simulink model "backbone"  (R2022b)
settings: Solver=FixedStepDiscrete  StartTime=0.0  StopTime=2  FixedStep=0.000001  RelTol=1e-3
undefined symbols (not defined in the file or in its folder): DiscIntNeverNeededParam, flux, Motor_flux, Motor_Ld_Indctances, Motor_Lq_Indctances, Motor_Pn, Motor_Rs, Pn, switch_electronic_feedworward, Switch_SubsysCtrl, SysCurrentMax, SysVoltage, Ts
libraries: powerlib_extras x11, simulink x4, mcbcontrolslib x4, slpidlib x3, spsPermanentMagnetSynchronousMachineLib x2, spsDCVoltageSourceLib x2, spsGroundLib x1, eePmsmCurrentController x1, spsThreePhaseVIMeasurementLib x1, spsTwoLevelConverterLib x1, spsUniversalBridgeLib x1, spspowerguiLib x1
(part 1 of 3)
settings Model: DataDictionary=modelDictionary.sldd  PacingRate=0.018000  Creator=yll  LastModifiedBy=yll

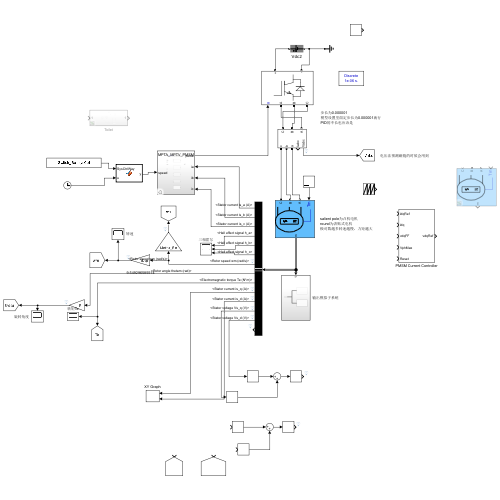
[thumbnail: Simulink's stored preview of the top-level diagram]
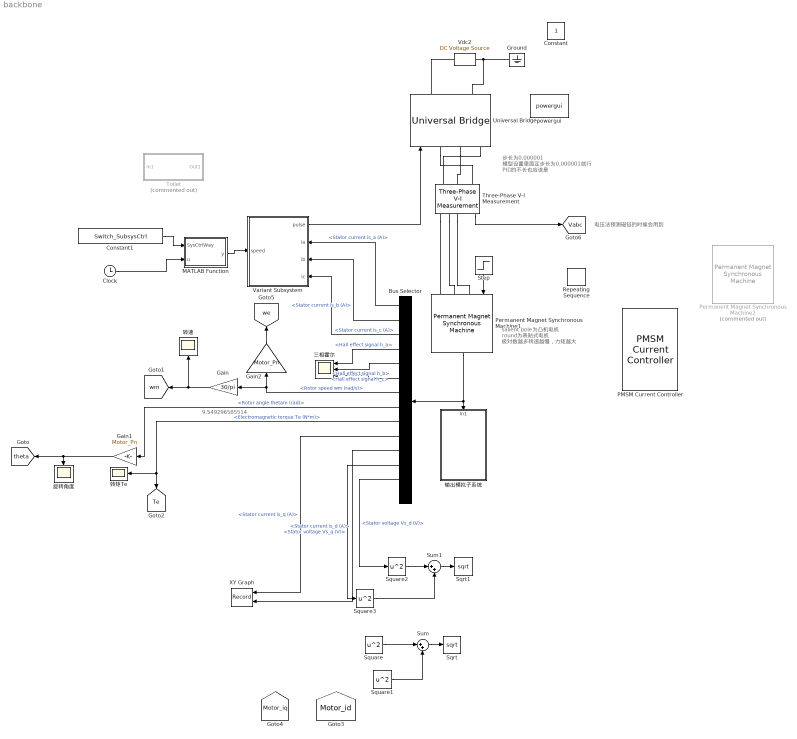
== system backbone ==
  note: 9.549296585514
  note: 电压法预测磁链的时候会用到
  note: salient pole为凸机电机
      | round为表贴式电机
      | 极对数越多转速越慢，力矩越大
  note: 步长为0.000001
      | 模型设置里面定步长为0.000001就行
      | PID的不长也应该是
  Bus Selector : BusSelector  OutputSignals=Stator current is_a (A),Stator current is_b (A),Stator current is_c (A),Hall effect signal h_a,Hall effect signal h_b,Hall effect signal h_c,Rotor speed wm (rad/s),Rotor angle thetam (rad),Electromagnetic torque Te (N*m),Stator current is_q (A),Stator current is_d (A),Stator voltage Vs_q (V),Stator voltage Vs_d (V),Electromagnetic torque Te (N*m)
  Clock : Clock
  Constant : Constant
  Constant1 : Constant  Value=Switch_SubsysCtrl
  Gain : Gain  Gain=30/pi
  Gain1 : Gain  Gain=Motor_Pn
  Gain2 : Gain  Gain=Motor_Pn
  Ground : spsGroundLib/Ground  LConnTagsString=a
  MATLAB Function : MATLAB Function  TreatAsAtomicUnit=on
  PMSM Current Controller : eePmsmCurrentController/PMSM Current Controller  Kp_id=1  Ki_id=100  Kaw_id=1  Kp_iq=1  Ki_iq=100  Kaw_iq=1  Ts=-1  Tsd=0.001  AxisPrio=Q-axis  ActZC=off  ActFF=on
      settings: LibrarySourceBlock=ee_sl_lib/PMSM Control/PMSM Current Controller
  Permanent Magnet Synchronous Machine1 : spsPermanentMagnetSynchronousMachineLib/Permanent Magnet Synchronous Machine  NbPhases=3  FluxDistribution=Sinusoidal  RotorType=Salient-pole  MechanicalLoad=Torque Tm  PresetModel=No  ShowDetailedParameters=on  MeasurementBus=off  Resistance=Motor_Rs  Inductance=8.5e-3  dqInductances=[Motor_Ld_Indctances Motor_Lq_Indctances]  La=Motor_Ld_Indctances  MachineConstant=Flux linkage established by magnets (V.s)  Flux=Motor_flux  VoltageCst=58.0416  TorqueCst=0.48  Flat=120  Mechanical=[0.003 0.008 Motor_Pn 0]  PolePairs=4  InitialConditions=[0,0, 0,0]  InitialConditions5ph=[0 0 0 0 0 0]  RefAngle=Aligned with phase A axis (original Park)  IterativeDiscreteModel=Trapezoidal robust  TsBlock=-1  TsPowergui=0
  Permanent Magnet Synchronous Machine2 : spsPermanentMagnetSynchronousMachineLib/Permanent Magnet Synchronous Machine  Commented=on  NbPhases=3  FluxDistribution=Sinusoidal  RotorType=Salient-pole  MechanicalLoad=Torque Tm  PresetModel=No  ShowDetailedParameters=on  MeasurementBus=off  Resistance=Motor_Rs  Inductance=8.5e-3  dqInductances=[Motor_Ld_Indctances Motor_Lq_Indctances]  La=Motor_Ld_Indctances  MachineConstant=Flux linkage established by magnets (V.s)  Flux=Motor_flux  VoltageCst=58.0416  TorqueCst=0.48  Flat=120  Mechanical=[0.003 0.008 Motor_Pn 0]  PolePairs=2  InitialConditions=[0,0, 0,0]  InitialConditions5ph=[0 0 0 0 0 0]  RefAngle=Aligned with phase A axis (original Park)  IterativeDiscreteModel=Trapezoidal robust  TsBlock=-1  TsPowergui=0
  Repeating Sequence : simulink/Sources/Repeating Sequence  rep_seq_t=[0 0.6 3]  rep_seq_y=[0 10 55.97]
  Sqrt : Sqrt
  Sqrt1 : Sqrt
  Square{,1..3} (4 alike) : Math  Operator=square
  Step : Step  Time=0.3  After=0  SampleTime=0
  Sum : Sum  Inputs=|++
  Sum1 : Sum  Inputs=|++
  Three-Phase V-I Measurement : spsThreePhaseVIMeasurementLib/Three-Phase V-I Measurement  VoltageMeasurement=phase-to-ground  SetLabelV=off  LabelV=Vabc  Vpu=off  VpuLL=off  CurrentMeasurement=yes  SetLabelI=off  LabelI=Iabc  Ipu=off  Pbase=100e6  Vbase=500e3  OutputType=Complex  PhasorSimulation=off  PSBequivalent=0
  Toilet : Subsystem  Commented=on
  Universal Bridge : spsUniversalBridgeLib/Universal Bridge  Arms=3  SnubberResistance=1e5  SnubberCapacitance=inf  Device=IGBT / Diodes  Ron=1e-3  Lon=0  ForwardVoltages="[  0  0  ]"  ForwardVoltage="[  0  0  ]"  GTOparameters=[ 10e-6 , 20e-6 ]  IGBTparameters=[ 1e-6 , 2e-6 ]  Measurements=None  Measurements_2=None  converterType=Rectifier
  Variant Subsystem : Subsystem  Variant=on
      settings: PortSchema="{\"entries\":[{\"content\":{\"sides\":[{\"content\":{\"connectorIds\":[\"In1\"]},\"type\":\"ConnectorPlacement.EquallySpacedRectSide\",\"uuid\":\"2e7849e6-0e6b-4177-ab4c-005e62b7a995\"},{\"content\":{\"connectorIds\":[\"Out1\",\"In2\",\"In3\",\"In4\"],\"side\":\"RIGHT\"},\"type\":\"ConnectorPlacement.EquallySpacedRectSide\",\"uuid\":\"63557eec-d5b5-4e2f-88ae-a2d5548ecb78\"},{\"content\":{\"connectorIds\":[],\"side\":\"TOP\"},\"type\":\"ConnectorPlacement.EquallySpacedRectSide\",\"uuid\":\"e5c96169-075b-4d07-a86b-1ba058334d10\"},{\"content\":{\"connectorIds\":[],\"side\":\"BOTTOM\"},\"type\":\"ConnectorPlacement.EquallySpacedRectSide\",\"uuid\":\"b7265cdc-8287-40f1-b4fb-8314bb99ac7b\"}]},\"type\":\"ConnectorPlacement.EquallySpacedConnector\",\"uuid\":\"3f47df4e-4e26-4395-afee-aeddf8227fe9\"}],\"packageUris\":[\"http://schema.mathworks.com/mf0/Connector/R2020b\"],\"version\":\"1.0\"}"
  Vdc2 : spsDCVoltageSourceLib/DC Voltage Source  Amplitude=SysVoltage  Measurements=None
  XY Graph : Record  FileSettingsInternal="{\"entries\":[{\"content\":{\"excelSettings\":{\"content\":{},\"type\":\"Streamout.ExcelSettings\"}},\"type\":\"Streamout.FileSettingStorage\",\"uuid\":\"9a52813c-0e76-4145-8ec9-bed97980991f\"}],\"packageUris\":[\"http://schema.mathworks.com/mf0/streamout_blocks/R2020a\"],\"version\":\"1.0\"}"  Layout=[1 1]  SignalsInternal="{\"entries\":[{\"content\":{\"signals\":[{\"content\":{\"blockPath\":[\"backbone/XY Graph\"],\"channel\":[],\"dimensions\":[1],\"domain\":\"backbone/XY Graph\",\"lineColor\":\"#a2142f\",\"plots\":[1],\"port\":1,\"sid\":[\"\"],\"signalID\":8996,\"signalName\":\"<Stator current is_q (A)>\"},\"type\":\"RecordBlkView.Signal\",\"uuid\":\"e11d3486-c8d0-4833-b26e-8d9d061e6f7c\"},{\"content\":{\"blockPath\":[\"backbone/XY Graph\"],\"channel\":[],\"dimensions\":[1],\"domain\":\"backbone/XY Graph\",\"lineColor\":\"#139fff\",\"plots\":[1],\"port\":2,\"sid\":[\"\"],\"signalID\":9000,\"signalName\":\"<Stator current is_d (A)>\"},\"type\":\"RecordBlkView.Signal\",\"uuid\":\"b0f723db-f625-4e0b-a689-0f7f588f8e97\"}]},\"type\":\"RecordBlkView.InputSignals\",\"uuid\":\"73730b23-746f-4a99-9d4b-303219e85664\"}],\"packageUris\":[\"http://schema.mathworks.com/mf0/streamout_blocks/R2020a\"],\"version\":\"1.0\"}"  VisualizationBindings="{\"xyplotplugin\":{\"info\":[{\"series\":[{\"bindingParametersList\":[{\"parameter\":\"X-Axis\",\"signalID\":8996,\"signalName\":\"<Stator current is_q (A)>\"},{\"parameter\":\"Y-Axis\",\"signalID\":9000,\"signalName\":\"<Stator current is_d (A)>\"}],\"seriesID\":62565}],\"subplotID\":1}]}}"  CompatibilityTag=XY
  powergui : spspowerguiLib/powergui  Priority=1  SimulationMode=Discrete  SampleTime=1e-6  frequency=60  Iterations=50  frequencyindice=0  Pbase=100e6  ErrMax=1e-4  UnitsV=kV  UnitsW=MW  buscounter=0  FunctionMessages=off  echomessages=off  EnableUseOfTLC=off  CurrentSourceSwitches=off  DisableSnubberDevices=off  DisableRonSwitches=off  DisableVfSwitches=off  DisplayEquations=off  AutomaticDiscreteSolvers=off  SolverType=Tustin/Backward Euler (TBE)  Interpol=off  ExternalGateDelay=off  methode=off  Ts=10  x0status=blocks  SPID=off  SwTol=0  HookPort=off  NonlinearTolerance=1e-4  nMaxIteration=100  ContinueOnMaxIteration=off  RestoreLinks=warning  ResistiveCurrentMeasurement=off  Frange=[0:2:500]  Ylog=off  Xlog=on  ShowGrid=off  save=off  variable=ZData  structure=current_abc  ZoomFFT=off  StartTime=0.1  cycles=1  DisplayStyle=1  fundamental=1  FreqAxis=off  MaxFrequency=100  frequencyindicesteady=1  RmsSteady=1  display=off
  三相霍尔 : Scope  NumInputPorts=3
  旋转角度 : Scope
  转矩Te : Scope
  转速 : Scope
  输出模拟子系统 : Subsystem
  tag scope: Motor_id=global, Motor_iq=global, Te=global, Vabc=global, theta=global, we=global, wm=global
  wires:
  Gain1/1 -> 旋转角度/1, [theta]
  Bus Selector/6 -> 三相霍尔/3  "<Hall effect signal h_c>"
  Bus Selector/4 -> 三相霍尔/1  "<Hall effect signal h_a>"
  Bus Selector/5 -> 三相霍尔/2  "<Hall effect signal h_b>"
  Gain/1 -> [wm], 转速/1
  Bus Selector/8 -> Gain1/1  "<Rotor angle thetam (rad)>"
  Bus Selector/7 -> Gain2/1, Gain/1  "<Rotor speed wm (rad/s)>"
  Permanent Magnet Synchronous Machine1/1 -> Bus Selector/1, 输出模拟子系统/1(In1)
  Variant Subsystem/1(pulse) -> Universal Bridge/1
  Gain2/1 -> [we]
  Three-Phase V-I Measurement/1 -> [Vabc]
  Bus Selector/9 -> [Te], 转矩Te/1  "<Electromagnetic torque Te (N*m)>"
  Bus Selector/1 -> Variant Subsystem/2(ia)  "<Stator current is_a (A)>"
  Bus Selector/2 -> Variant Subsystem/3(ib)  "<Stator current is_b (A)>"
  Bus Selector/3 -> Variant Subsystem/4(ic)  "<Stator current is_c (A)>"
  Square/1 -> Sum/1
  Square1/1 -> Sum/2
  Sum/1 -> Sqrt/1
  Square2/1 -> Sum1/1
  Sum1/1 -> Sqrt1/1
  Square3/1 -> Sum1/2
  Bus Selector/12 -> Square3/1  "<Stator voltage Vs_q (V)>"
  Bus Selector/13 -> Square2/1  "<Stator voltage Vs_d (V)>"
  Step/1 -> Permanent Magnet Synchronous Machine1/1
  Bus Selector/10 -> XY Graph/1  "<Stator current is_q (A)>"
  Bus Selector/11 -> XY Graph/2  "<Stator current is_d (A)>"
  Clock/1 -> MATLAB Function/2(u)
  MATLAB Function/1(y) -> Variant Subsystem/1(speed)
  Constant1/1 -> MATLAB Function/1(SysCtrlWay)
  connections:
  Vdc2/RConn1 -- Universal Bridge/RConn1
  Vdc2/LConn1 -- Universal Bridge/RConn2 -- Ground/LConn1
  Universal Bridge/LConn1 -- Three-Phase V-I Measurement/LConn1
  Universal Bridge/LConn2 -- Three-Phase V-I Measurement/LConn2
  Universal Bridge/LConn3 -- Three-Phase V-I Measurement/LConn3
  Three-Phase V-I Measurement/RConn1 -- Permanent Magnet Synchronous Machine1/LConn1
  Three-Phase V-I Measurement/RConn2 -- Permanent Magnet Synchronous Machine1/LConn2
  Three-Phase V-I Measurement/RConn3 -- Permanent Magnet Synchronous Machine1/LConn3

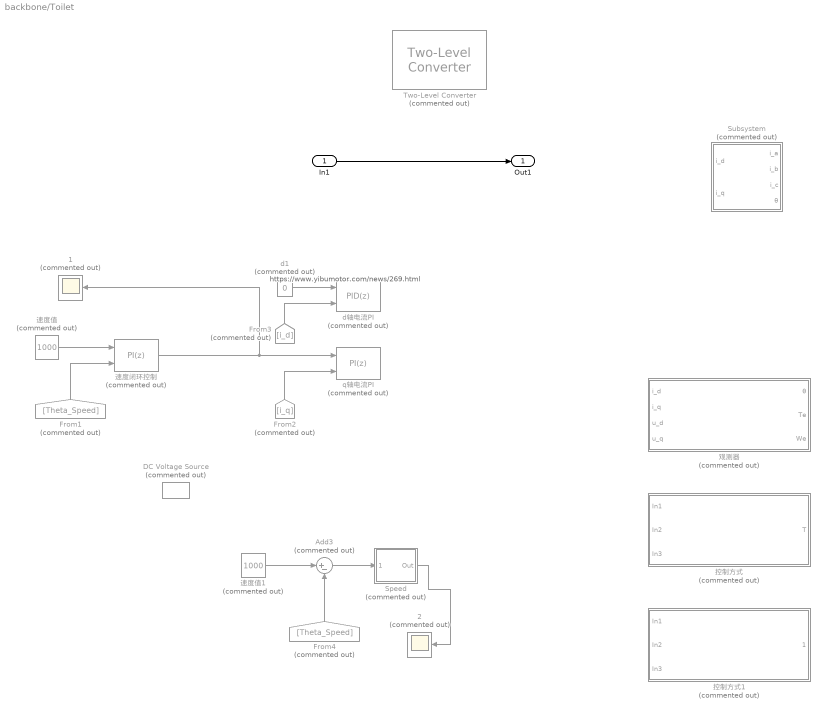
== system backbone/Toilet ==
  note: https://www.yibumotor.com/news/269.html
  In1 : Inport
  " 1" : Scope  Commented=on
  " 2" : Scope  Commented=on
  Add3 : Sum  Commented=on  Inputs=|+-
  DC Voltage Source : spsDCVoltageSourceLib/DC Voltage Source  Commented=on  Amplitude=311  Measurements=None
  From1 : From  Commented=on  GotoTag=Theta_Speed
  From2 : From  Commented=on  GotoTag=i_q
  From3 : From  Commented=on  GotoTag=i_d
  From4 : From  Commented=on  GotoTag=Theta_Speed
  Speed : Subsystem  Commented=on  AncestorBlock=|  DialogController=POWERSYS.PowerSysDialog  mask(Discrete PI Controller){C=1, Mu=1, q=200, Par_Limits=[1000 -1000], Init=0, Ts=0.000001}
      | powerlib_extras/Discrete 
      | Control Blocks/Discrete
      | PI Controller
      mask prompts: C "Gain (c):"; Mu "Gain (Mu):"; q "Gain (q)"; Par_Limits "Output limits: [ Upper   Lower ]"; Init "Output initial value:"; Ts "Sample time:"
      mask help: This block implements a discrete PI controller.
      mask init:
      | UpperLimit=Par_Limits(1);
      | LowerLimit=Par_Limits(2);
      | power_initmask();
      settings: LibrarySourceBlock=|
      | powerlib_extras/Discrete
      | Control Blocks/Discrete
      | PI Controller
      mask Help: This block is part of a subset of blocks in the Extras library that does not have documentation associated with it, other than the block mask description.
      mask Display: disp('SMC');
  Subsystem : Subsystem  Commented=on
  Two-Level Converter : spsTwoLevelConverterLib/Two-Level Converter  Commented=on  ModelType=Switching devices  Ron=1e-3  Rs=1e6  Cs=inf  Vforward=[0,0]  Ron_Diode=1e-3  Rs_Diode=1e6  Cs_Diode=inf  Vf_Diode=1e-3  Rs_CurrentSource=inf  Ron_ACsource=1e-3
      settings: LibrarySourceBlock=sps_lib/Power Electronics/Two-Level Converter
  d1 : Constant  Commented=on  Value=0
  d轴电流PI : slpidlib/PID Controller (2DOF)  Commented=on  Controller=PID  Form=Parallel  TimeDomain=Discrete-time  UseExternalTs=off  SampleTime=-1  IntegratorMethod=Forward Euler  FilterMethod=Forward Euler  ControllerParametersSource=internal  P=16.4  I=5750  UseKiTs=off  D=0  N=100  UseFilter=on  b=1  c=1  TunerSelectOption=Transfer Function Based (PID Tuner App)  InitialConditionSource=internal  InitialConditionForIntegrator=0  InitialConditionForFilter=0  DifferentiatorICPrevScaledInput=0  ExternalReset=none  TrackingMode=off  Kt=1  LimitOutput=off  SatLimitsSource=internal  UpperSaturationLimit=inf  LowerSaturationLimit=-inf  LinearizeAsGain=off  AntiWindupMode=none  Kb=1  LimitIntegrator=off  UpperIntegratorSaturationLimit=inf  LowerIntegratorSaturationLimit=-inf  POutMin=[]  POutMax=[]  IOutMin=[]  IOutMax=[]  DOutMin=[]  DOutMax=[]  NOutMin=[]  NOutMax=[]  bOutMin=[]  bOutMax=[]  cOutMin=[]  cOutMax=[]  SumOutMin=[]  SumOutMax=[]  SaturationOutMin=[]  SaturationOutMax=[]  PParamMin=[]  PParamMax=[]  IParamMin=[]  IParamMax=[]  DParamMin=[]  DParamMax=[]  NParamMin=[]  NParamMax=[]  bParamMin=[]  bParamMax=[]  cParamMin=[]  cParamMax=[]  KbParamMin=[]  KbParamMax=[]  KtParamMin=[]  KtParamMax=[]  KbOutMin=[]  KbOutMax=[]  KtOutMin=[]  KtOutMax=[]  IntegratorOutMin=[]  IntegratorOutMax=[]  FilterOutMin=[]  FilterOutMax=[]  SumI1OutMin=[]  SumI1OutMax=[]  SumI2OutMin=[]  SumI2OutMax=[]  SumI3OutMin=[]  SumI3OutMax=[]  SumI4OutMin=[]  SumI4OutMax=[]  SumDOutMin=[]  SumDOutMax=[]  Sum1OutMin=[]  Sum1OutMax=[]  Sum2OutMin=[]  Sum2OutMax=[]  Sum3OutMin=[]  Sum3OutMax=[]  DifferentiatorOutMin=[]  DifferentiatorOutMax=[]  FilterDiffOutCoefMin=[]  FilterDiffOutCoefMax=[]  ReciprocalOutMin=[]  ReciprocalOutMax=[]  SumDenOutMin=[]  SumDenOutMax=[]  SumNumOutMin=[]  SumNumOutMax=[]  DivideOutMin=[]  DivideOutMax=[]  UdiffTsProdOutMin=[]  UdiffTsProdOutMax=[]  NTsProdOutMin=[]  NTsProdOutMax=[]  UintegralTsProdOutMin=[]  UintegralTsProdOutMax=[]  UngainTsProdOutMin=[]  UngainTsProdOutMax=[]  ClampingZeroOutDataTypeStr=Inherit: Inherit via back propagation  ClampingZeroOutMin=[]  ClampingZeroOutMax=[]  FilterDenConstantOutDataTypeStr=Inherit: Inherit via back propagation  FilterDenConstantOutMin=[]  FilterDenConstantOutMax=[]  PCopyOutDataTypeStr=Inherit: Inherit via back propagation  PCopyOutMin=[]  PCopyOutMax=[]  NCopyOutDataTypeStr=Inherit: Inherit via back propagation  NCopyOutMin=[]  NCopyOutMax=[]  IntegratorContinuousStateAttributes=''  IntegratorStateMustResolveToSignalObject=off  IntegratorRTWStateStorageClass=Auto  FilterContinuousStateAttributes=''  FilterStateMustResolveToSignalObject=off  FilterRTWStateStorageClass=Auto  ParallelPVariant=InternalParameters  IdealPVariant=Disabled  IVariant=InternalParameters  DVariant=InternalParameters  bVariant=InternalParameters  cVariant=InternalParameters  IntegratorVariant=Discrete  SatVariant=Disabled  AWVariant=Passthrough  PCopyVariant=Disabled  TRVariant=Disabled  FdbkBlocksVariant=Forward  IdealPFdbkVariant=Disabled  SatFdbkVariant=Disabled  DerivativeFilterVariant=ForwardEulerFilter  NVariant=InternalParameters  NCopyVariant=Disabled  FilterICVariant=InternalICsFilter  IntegratorICVariant=InternalICs  ExternalResetVariant=Disabled  TRSumVariant=Passthrough  SumFdbkVariant=Disabled  SumVariant=Sum_PID  TsampFilterVariant=InternalTs  TsampNgainVariant=Passthrough  TsampIntegralVariant=Passthrough  ExternalSaturationOutDataTypeStr=Inherit: Same as second input
  q轴电流PI : slpidlib/PID Controller (2DOF)  Commented=on  Controller=PI  Form=Parallel  TimeDomain=Discrete-time  UseExternalTs=off  SampleTime=0.000001  IntegratorMethod=Forward Euler  FilterMethod=Forward Euler  ControllerParametersSource=internal  P=16.4  I=5750  UseKiTs=off  D=0  N=100  UseFilter=on  b=1  c=1  TunerSelectOption=Transfer Function Based (PID Tuner App)  InitialConditionSource=internal  InitialConditionForIntegrator=0  InitialConditionForFilter=0  DifferentiatorICPrevScaledInput=0  ExternalReset=none  TrackingMode=off  Kt=1  LimitOutput=off  SatLimitsSource=internal  UpperSaturationLimit=inf  LowerSaturationLimit=-inf  LinearizeAsGain=off  AntiWindupMode=none  Kb=1  LimitIntegrator=off  UpperIntegratorSaturationLimit=inf  LowerIntegratorSaturationLimit=-inf  POutMin=[]  POutMax=[]  IOutMin=[]  IOutMax=[]  DOutMin=[]  DOutMax=[]  NOutMin=[]  NOutMax=[]  bOutMin=[]  bOutMax=[]  cOutMin=[]  cOutMax=[]  SumOutMin=[]  SumOutMax=[]  SaturationOutMin=[]  SaturationOutMax=[]  PParamMin=[]  PParamMax=[]  IParamMin=[]  IParamMax=[]  DParamMin=[]  DParamMax=[]  NParamMin=[]  NParamMax=[]  bParamMin=[]  bParamMax=[]  cParamMin=[]  cParamMax=[]  KbParamMin=[]  KbParamMax=[]  KtParamMin=[]  KtParamMax=[]  KbOutMin=[]  KbOutMax=[]  KtOutMin=[]  KtOutMax=[]  IntegratorOutMin=[]  IntegratorOutMax=[]  FilterOutMin=[]  FilterOutMax=[]  SumI1OutMin=[]  SumI1OutMax=[]  SumI2OutMin=[]  SumI2OutMax=[]  SumI3OutMin=[]  SumI3OutMax=[]  SumI4OutMin=[]  SumI4OutMax=[]  SumDOutMin=[]  SumDOutMax=[]  Sum1OutMin=[]  Sum1OutMax=[]  Sum2OutMin=[]  Sum2OutMax=[]  Sum3OutMin=[]  Sum3OutMax=[]  DifferentiatorOutMin=[]  DifferentiatorOutMax=[]  FilterDiffOutCoefMin=[]  FilterDiffOutCoefMax=[]  ReciprocalOutMin=[]  ReciprocalOutMax=[]  SumDenOutMin=[]  SumDenOutMax=[]  SumNumOutMin=[]  SumNumOutMax=[]  DivideOutMin=[]  DivideOutMax=[]  UdiffTsProdOutMin=[]  UdiffTsProdOutMax=[]  NTsProdOutMin=[]  NTsProdOutMax=[]  UintegralTsProdOutMin=[]  UintegralTsProdOutMax=[]  UngainTsProdOutMin=[]  UngainTsProdOutMax=[]  ClampingZeroOutDataTypeStr=Inherit: Inherit via back propagation  ClampingZeroOutMin=[]  ClampingZeroOutMax=[]  FilterDenConstantOutDataTypeStr=Inherit: Inherit via back propagation  FilterDenConstantOutMin=[]  FilterDenConstantOutMax=[]  PCopyOutDataTypeStr=Inherit: Inherit via back propagation  PCopyOutMin=[]  PCopyOutMax=[]  NCopyOutDataTypeStr=Inherit: Inherit via back propagation  NCopyOutMin=[]  NCopyOutMax=[]  IntegratorContinuousStateAttributes=''  IntegratorStateMustResolveToSignalObject=off  IntegratorRTWStateStorageClass=Auto  FilterContinuousStateAttributes=''  FilterStateMustResolveToSignalObject=off  FilterRTWStateStorageClass=Auto  ParallelPVariant=InternalParameters  IdealPVariant=Disabled  IVariant=InternalParameters  DVariant=Disabled  bVariant=InternalParameters  cVariant=Disabled  IntegratorVariant=Discrete  SatVariant=Disabled  AWVariant=Passthrough  PCopyVariant=Disabled  TRVariant=Disabled  FdbkBlocksVariant=Forward  IdealPFdbkVariant=Disabled  SatFdbkVariant=Disabled  DerivativeFilterVariant=Disabled  NVariant=Disabled  NCopyVariant=Disabled_SignalSpec  FilterICVariant=Disabled  IntegratorICVariant=InternalICs  ExternalResetVariant=Disabled  TRSumVariant=Passthrough  SumFdbkVariant=Disabled  SumVariant=Sum_PI  TsampFilterVariant=InternalTs  TsampNgainVariant=Passthrough  TsampIntegralVariant=Passthrough  ExternalSaturationOutDataTypeStr=Inherit: Same as second input
  控制方式 : Subsystem  Commented=on  Variant=on
  控制方式1 : Subsystem  Commented=on  Variant=on
  观测器 : Subsystem  Commented=on  Variant=on
  速度值 : Constant  Commented=on  Value=1000
  速度值1 : Constant  Commented=on  Value=1000
  速度闭环控制 : slpidlib/PID Controller (2DOF)  Commented=on  Controller=PI  Form=Parallel  TimeDomain=Discrete-time  UseExternalTs=off  SampleTime=0.000001  IntegratorMethod=Forward Euler  FilterMethod=Forward Euler  ControllerParametersSource=internal  P=0.7  I=5  UseKiTs=off  D=0  N=100  UseFilter=on  b=1  c=1  TunerSelectOption=Transfer Function Based (PID Tuner App)  InitialConditionSource=internal  InitialConditionForIntegrator=0  InitialConditionForFilter=0  DifferentiatorICPrevScaledInput=0  ExternalReset=none  TrackingMode=off  Kt=1  LimitOutput=off  SatLimitsSource=internal  UpperSaturationLimit=inf  LowerSaturationLimit=-inf  LinearizeAsGain=off  AntiWindupMode=none  Kb=1  LimitIntegrator=off  UpperIntegratorSaturationLimit=inf  LowerIntegratorSaturationLimit=-inf  POutMin=[]  POutMax=[]  IOutMin=[]  IOutMax=[]  DOutMin=[]  DOutMax=[]  NOutMin=[]  NOutMax=[]  bOutMin=[]  bOutMax=[]  cOutMin=[]  cOutMax=[]  SumOutMin=[]  SumOutMax=[]  SaturationOutMin=[]  SaturationOutMax=[]  PParamMin=[]  PParamMax=[]  IParamMin=[]  IParamMax=[]  DParamMin=[]  DParamMax=[]  NParamMin=[]  NParamMax=[]  bParamMin=[]  bParamMax=[]  cParamMin=[]  cParamMax=[]  KbParamMin=[]  KbParamMax=[]  KtParamMin=[]  KtParamMax=[]  KbOutMin=[]  KbOutMax=[]  KtOutMin=[]  KtOutMax=[]  IntegratorOutMin=[]  IntegratorOutMax=[]  FilterOutMin=[]  FilterOutMax=[]  SumI1OutMin=[]  SumI1OutMax=[]  SumI2OutMin=[]  SumI2OutMax=[]  SumI3OutMin=[]  SumI3OutMax=[]  SumI4OutMin=[]  SumI4OutMax=[]  SumDOutMin=[]  SumDOutMax=[]  Sum1OutMin=[]  Sum1OutMax=[]  Sum2OutMin=[]  Sum2OutMax=[]  Sum3OutMin=[]  Sum3OutMax=[]  DifferentiatorOutMin=[]  DifferentiatorOutMax=[]  FilterDiffOutCoefMin=[]  FilterDiffOutCoefMax=[]  ReciprocalOutMin=[]  ReciprocalOutMax=[]  SumDenOutMin=[]  SumDenOutMax=[]  SumNumOutMin=[]  SumNumOutMax=[]  DivideOutMin=[]  DivideOutMax=[]  UdiffTsProdOutMin=[]  UdiffTsProdOutMax=[]  NTsProdOutMin=[]  NTsProdOutMax=[]  UintegralTsProdOutMin=[]  UintegralTsProdOutMax=[]  UngainTsProdOutMin=[]  UngainTsProdOutMax=[]  ClampingZeroOutDataTypeStr=Inherit: Inherit via back propagation  ClampingZeroOutMin=[]  ClampingZeroOutMax=[]  FilterDenConstantOutDataTypeStr=Inherit: Inherit via back propagation  FilterDenConstantOutMin=[]  FilterDenConstantOutMax=[]  PCopyOutDataTypeStr=Inherit: Inherit via back propagation  PCopyOutMin=[]  PCopyOutMax=[]  NCopyOutDataTypeStr=Inherit: Inherit via back propagation  NCopyOutMin=[]  NCopyOutMax=[]  IntegratorContinuousStateAttributes=''  IntegratorStateMustResolveToSignalObject=off  IntegratorRTWStateStorageClass=Auto  FilterContinuousStateAttributes=''  FilterStateMustResolveToSignalObject=off  FilterRTWStateStorageClass=Auto  ParallelPVariant=InternalParameters  IdealPVariant=Disabled  IVariant=InternalParameters  DVariant=Disabled  bVariant=InternalParameters  cVariant=Disabled  IntegratorVariant=Discrete  SatVariant=Disabled  AWVariant=Passthrough  PCopyVariant=Disabled  TRVariant=Disabled  FdbkBlocksVariant=Forward  IdealPFdbkVariant=Disabled  SatFdbkVariant=Disabled  DerivativeFilterVariant=Disabled  NVariant=Disabled  NCopyVariant=Disabled_SignalSpec  FilterICVariant=Disabled  IntegratorICVariant=InternalICs  ExternalResetVariant=Disabled  TRSumVariant=Passthrough  SumFdbkVariant=Disabled  SumVariant=Sum_PI  TsampFilterVariant=InternalTs  TsampNgainVariant=Passthrough  TsampIntegralVariant=Passthrough  ExternalSaturationOutDataTypeStr=Inherit: Same as second input
  Out1 : Outport
  wires:
  In1/1 -> Out1/1
  From2/1 -> q轴电流PI/2
  d1/1 -> d轴电流PI/1
  From4/1 -> Add3/2
  From1/1 -> 速度闭环控制/2
  From3/1 -> d轴电流PI/2
  速度闭环控制/1 -> q轴电流PI/1, " 1"/1
  速度值1/1 -> Add3/1
  Add3/1 -> Speed/1(Error)
  速度值/1 -> 速度闭环控制/1
  Speed/1(Out) -> " 2"/1

== system backbone/Variant Subsystem ==
  note: 1) Add Subsystem or Model blocks as valid variant choices.
      | 2) You cannot connect blocks at this level. At simulation, connectivity is automatically
      | determined, based on the active variant and port name matching.
  speed : Inport
  ia : Inport  Port=2
  ib : Inport  Port=3
  ic : Inport  Port=4
  BangBang_PMSM : Subsystem  VariantControl=Switch_SubsysCtrl==2
  DTC_PMSM : Subsystem  VariantControl=Switch_SubsysCtrl==3
  DTC_SVPWM_PMSM : Subsystem  VariantControl=Switch_SubsysCtrl==4
  MPTA_MPTV_PMSM : Subsystem  VariantControl=Switch_SubsysCtrl==5
  SMC_OR_PID : Subsystem  VariantControl=Switch_SubsysCtrl==0|Switch_SubsysCtrl==1
  pulse : Outport

== system backbone/输出模拟子系统 ==
  In1 : Inport
  clark和park变换模拟 : Subsystem  Commented=on
  磁链模拟 : Subsystem
  wires:
  In1/1 -> 磁链模拟/1(In1), clark和park变换模拟/1(In1)

== system backbone/Toilet/Speed ==
  Error : Inport  SampleTime=Ts
  1/D : Gain  Gain=1/(1.5*Pn*flux/0.003)  SaturateOnIntegerOverflow=on  SampleTime=Ts  OutDataTypeStr=Inherit: Same as input  ParamDataTypeStr=Inherit: Same as input
  Discrete Derivative : simulink/Discrete/Discrete Derivative  gainval=1.0  ICPrevScaledInput=0.0  OutMin=[]  OutMax=[]  OutDataType=fixdt(1, 16)  OutScaling=2^-10  DoSatur=off
  Discrete-Time Integrator : DiscreteIntegrator  InitialCondition=0.001  SampleTime=Ts  ICPrevOutput=DiscIntNeverNeededParam  ICPrevScaledInput=DiscIntNeverNeededParam
  Kp1 : Gain  Gain=q  SaturateOnIntegerOverflow=on  SampleTime=Ts  OutDataTypeStr=Inherit: Same as input  ParamDataTypeStr=Inherit: Same as input
  Kp2 : Gain  Gain=Mu  SaturateOnIntegerOverflow=on  SampleTime=Ts  OutDataTypeStr=Inherit: Same as input  ParamDataTypeStr=Inherit: Same as input
  Kp3 : Gain  Gain=C  SaturateOnIntegerOverflow=on  SampleTime=Ts  OutDataTypeStr=Inherit: Same as input  ParamDataTypeStr=Inherit: Same as input
  Kp4 : Gain  Gain=C  SaturateOnIntegerOverflow=on  SampleTime=Ts  OutDataTypeStr=Inherit: Same as input  ParamDataTypeStr=Inherit: Same as input
  Nr->wm : Gain  Gain=pi/30  SaturateOnIntegerOverflow=on  SampleTime=Ts  OutDataTypeStr=Inherit: Same as input  ParamDataTypeStr=Inherit: Same as input
  Saturation2 : Saturate  UpperLimit=UpperLimit  LowerLimit=LowerLimit  SampleTime=Ts
  Sign : Signum
  Sum1 : Sum  InputSameDT=on  SaturateOnIntegerOverflow=on  SampleTime=Ts  OutDataTypeStr=Inherit: Same as first input
  Sum2 : Sum  Inputs=++-  InputSameDT=on  SaturateOnIntegerOverflow=on  SampleTime=Ts  OutDataTypeStr=Inherit: Same as first input
  Out : Outport  SampleTime=Ts  InitialOutput=0
  wires:
  Kp4/1 -> Sum1/1
  Saturation2/1 -> Out/1
  Discrete Derivative/1 -> Kp3/1, Sum1/2
  Sum2/1 -> Discrete-Time Integrator/1
  Error/1 -> Nr->wm/1
  Kp1/1 -> Sum2/1
  Sign/1 -> Kp2/1
  Sum1/1 -> Sign/1, Kp1/1
  Kp2/1 -> Sum2/2
  Kp3/1 -> Sum2/3
  1/D/1 -> Saturation2/1
  Discrete-Time Integrator/1 -> 1/D/1
  Nr->wm/1 -> Discrete Derivative/1, Kp4/1

== system backbone/Toilet/Subsystem ==
  i_a : Inport
  i_b : Inport  Port=2
  i_c : Inport  Port=3
  θ : Inport  Port=4
  Model : ModelReference  ModelNameDialog=ParkTran.slx  SimulationMode=Normal  ModelReferenceVersion=1.9
  Model1 : ModelReference  ModelNameDialog=ClarkTran.slx  SimulationMode=Normal  ModelReferenceVersion=1.13
  三相电流3 : Scope  NumInputPorts=3
  三相电流4 : Scope  NumInputPorts=2
  三相电流5 : Scope  NumInputPorts=2
  i_d : Outport
  i_q : Outport  Port=2
  wires:
  Model1/1 -> 三相电流4/1, Model/1
  i_b/1 -> Model1/2, 三相电流3/2
  Model1/2 -> 三相电流4/2, Model/2
  Model/1 -> i_d/1, 三相电流5/1
  Model/2 -> i_q/1, 三相电流5/2
  i_a/1 -> Model1/1, 三相电流3/1
  i_c/1 -> Model1/3, 三相电流3/3
  θ/1 -> Model/3

== system backbone/Toilet/控制方式 ==
  note: 1) Add Subsystem or Model blocks as valid variant choices.
      | 2) You cannot connect blocks at this level. At simulation, connectivity is automatically
      | determined, based on the active variant and port name matching.
  In1 : Inport
  In2 : Inport  Port=2
  In3 : Inport  Port=3
  DTC : ModelReference  ModelNameDialog=testmodel2.slx  VariantControl=true  ModelReferenceVersion=1.7
  FOC : ModelReference  DisableCoverage=on  ModelNameDialog=testmodel1.slx  VariantControl=false  ModelReferenceVersion=1.6
  T : Outport

== system backbone/Toilet/控制方式1 ==
  note: 1) Add Subsystem or Model blocks as valid variant choices.
      | 2) You cannot connect blocks at this level. At simulation, connectivity is automatically
      | determined, based on the active variant and port name matching.
  In1 : Inport
  In2 : Inport  Port=2
  In3 : Inport  Port=3
  PWM : ModelReference  DisableCoverage=on  ModelNameDialog=testmodel1.slx  VariantControl=false  ModelReferenceVersion=1.6
  SPWM : ModelReference  ModelNameDialog=testmodel2.slx  VariantControl=false  ModelReferenceVersion=1.7
  SVPWM : ModelReference  ModelNameDialog=testmodel2.slx  VariantControl=true  ModelReferenceVersion=1.7
  1 : Outport

== system backbone/Toilet/观测器 ==
  note: 1) Add Subsystem or Model blocks as valid variant choices.
      | 2) You cannot connect blocks at this level. At simulation, connectivity is automatically
      | determined, based on the active variant and port name matching.
  i_d : Inport
  i_q : Inport  Port=2
  u_d : Inport  Port=3
  u_q : Inport  Port=4
  Extended Kalman Filter : ModelReference  ModelNameDialog=testmodel2.slx  VariantControl=vm_Observer_Switch==2  ModelReferenceVersion=1.7
  Stationary coordinate system SMC αβ : ModelReference  ModelNameDialog=testmodel2.slx  VariantControl=vm_Observer_Switch==3  ModelReferenceVersion=1.7
  Synchronous rotating coordinate system SMC dq : ModelReference  DisableCoverage=on  ModelNameDialog=testmodel1.slx  VariantControl=vm_Observer_Switch==1  ModelReferenceVersion=1.6
  θ : Outport
  Te : Outport  Port=2
  We : Outport  Port=3

== system backbone/Variant Subsystem/BangBang_PMSM ==
  ia : Inport
  ib : Inport  Port=2
  ic : Inport  Port=3
  speed : Inport  Port=4
  Constant : Constant  Value=0
  Model1 : ModelReference  ModelNameDialog=InvParkTran.slx  SimulationMode=Normal  ModelReferenceVersion=1.8
  Model2 : ModelReference  ModelNameDialog=BangBang.slx  SimulationMode=Normal  ModelReferenceVersion=1.26
  Speed : Subsystem  AncestorBlock=|  DialogController=POWERSYS.PowerSysDialog  mask(Discrete PI Controller){Kpw=0.073, Kiw=0, Ba=0, Par_Limits=[50*sqrt(2) -50*sqrt(2)], Init=0, Ts=Ts}
      | powerlib_extras/Discrete 
      | Control Blocks/Discrete
      | PI Controller
      mask prompts: Kpw "Proportional gain (Kp):"; Kiw "Integral gain (Ki):"; Ba "feedback gain (Ba)"; Par_Limits "Output limits: [ Upper   Lower ]"; Init "Output initial value:"; Ts "Sample time:"
      mask help: This block implements a discrete PI controller.
      mask init:
      | UpperLimit=Par_Limits(1);
      | LowerLimit=Par_Limits(2);
      | power_initmask();
      settings: LibrarySourceBlock=|
      | powerlib_extras/Discrete
      | Control Blocks/Discrete
      | PI Controller
      mask Help: This block is part of a subset of blocks in the Extras library that does not have documentation associated with it, other than the block mask description.
      mask Display: disp('PI');
  Sum : Sum  Inputs=|+-
  pulse : Outport
  wires:
  speed/1 -> Sum/1
  [we] -> Sum/2
  Sum/1 -> Speed/1(Error)
  [theta] -> Model1/3
  ia/1 -> Model2/1
  ic/1 -> Model2/3
  ib/1 -> Model2/2
  Speed/1(Out) -> Model1/2
  Model1/1 -> Model2/4
  Model1/2 -> Model2/5
  Model2/1 -> pulse/1
  Constant/1 -> Model1/1

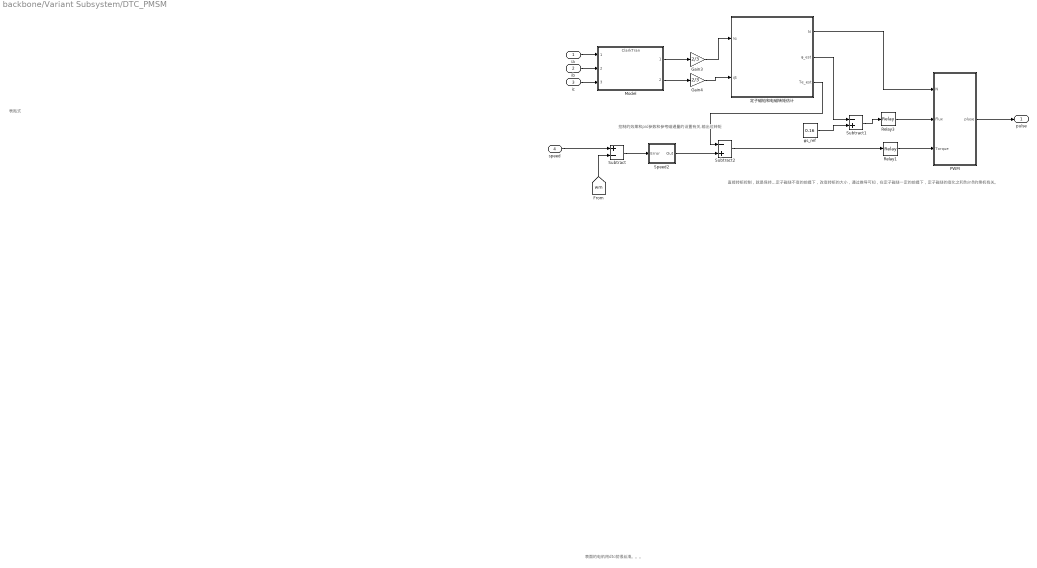
== system backbone/Variant Subsystem/DTC_PMSM ==
  note: 表贴式
  note: 控制的效果和pid参数和参考磁通量的设置有关,输出位转矩
  note: 直接转矩控制，就是保持定子磁链不变的前提下，改变转矩的大小，通过推导可知，在定子磁链一定的前提下，定子磁链的变化之和θsinθ的乘机有关。
  note: 表面的电机用dtc就很丝滑。。。
  ia : Inport
  ib : Inport  Port=2
  ic : Inport  Port=3
  speed : Inport  Port=4
  Gain3 : Gain  Gain=2/3
  Gain4 : Gain  Gain=2/3
  Model : ModelReference  ModelNameDialog=ClarkTran.slx  SimulationMode=Normal  ModelReferenceVersion=1.13
  PWM : Subsystem
  Relay1 : Relay  OnSwitchValue=0.00002  OffSwitchValue=-0.00002
  Relay3 : Relay  OnSwitchValue=0.00002  OffSwitchValue=-0.00002  InputProcessing=Columns as channels (frame based)
  Speed2 : Subsystem  AncestorBlock=|  DialogController=POWERSYS.PowerSysDialog  mask(Discrete PI Controller){Kpw=0.0114, Kiw=0.019, Ba=0, Par_Limits=[33.49 -33.49], Init=0, Ts=1e-6}
      | powerlib_extras/Discrete 
      | Control Blocks/Discrete
      | PI Controller
      mask prompts: Kpw "Proportional gain (Kp):"; Kiw "Integral gain (Ki):"; Ba "feedback gain (Ba)"; Par_Limits "Output limits: [ Upper   Lower ]"; Init "Output initial value:"; Ts "Sample time:"
      mask help: This block implements a discrete PI controller.
      mask init:
      | UpperLimit=Par_Limits(1);
      | LowerLimit=Par_Limits(2);
      | power_initmask();
      settings: LibrarySourceBlock=|
      | powerlib_extras/Discrete
      | Control Blocks/Discrete
      | PI Controller
      mask Help: This block is part of a subset of blocks in the Extras library that does not have documentation associated with it, other than the block mask description.
      mask Display: disp('PI');
  Subtract : Sum  Inputs=+-
  Subtract1 : Sum  Inputs=-+
  Subtract2 : Sum  Inputs=-+
  φs_ref : Constant  Value=0.16  VectorParams1D=off  SampleTime=Ts
  定子磁链和电磁转矩估计 : Subsystem  Variant=on
  pulse : Outport
  wires:
  ib/1 -> Model/2
  [wm] -> Subtract/2
  Relay1/1 -> PWM/3(Torque)
  Relay3/1 -> PWM/2(Flux)
  PWM/1(pluse) -> pulse/1
  Subtract1/1 -> Relay3/1
  φs_ref/1 -> Subtract1/2
  speed/1 -> Subtract/1
  Subtract2/1 -> Relay1/1
  定子磁链和电磁转矩估计/2(φ_est) -> Subtract1/1
  定子磁链和电磁转矩估计/1(N) -> PWM/1(N)
  ia/1 -> Model/1
  ic/1 -> Model/3
  定子磁链和电磁转矩估计/3(Te_est) -> Subtract2/1
  Speed2/1(Out) -> Subtract2/2
  Subtract/1 -> Speed2/1(Error)
  Model/2 -> Gain4/1
  Gain4/1 -> 定子磁链和电磁转矩估计/2(iβ)
  Model/1 -> Gain3/1
  Gain3/1 -> 定子磁链和电磁转矩估计/1(Iα)

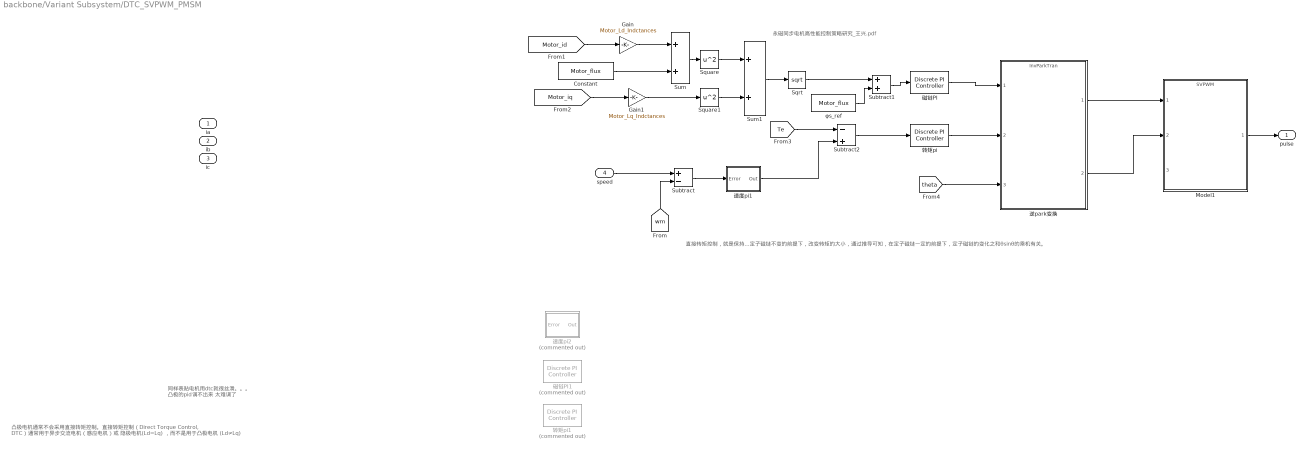
== system backbone/Variant Subsystem/DTC_SVPWM_PMSM ==
  note: 凸极电机通常不会采用直接转矩控制。直接转矩控制（Direct Torque Control, DTC）通常用于异步交流电机（感应电机）或 隐极电机(Ld=Lq) ，而不是用于凸极电机 (Ld≠Lq)
  note: 永磁同步电机高性能控制策略研究_王兴.pdf
  note: 直接转矩控制，就是保持定子磁链不变的前提下，改变转矩的大小，通过推导可知，在定子磁链一定的前提下，定子磁链的变化之和θsinθ的乘机有关。
  note: 同样表贴电机用dtc就很丝滑。。。
      | 凸极的pid调不出来 太难调了
  ia : Inport
  ib : Inport  Port=2
  ic : Inport  Port=3
  speed : Inport  Port=4
  Constant : Constant  Value=Motor_flux
  Gain : Gain  Gain=Motor_Ld_Indctances
  Gain1 : Gain  Gain=Motor_Lq_Indctances
  Model1 : ModelReference  ModelNameDialog=SVPWM.slx  SimulationMode=Normal  ModelReferenceVersion=1.9
  Sqrt : Sqrt
  Square : Math  Operator=square
  Square1 : Math  Operator=square
  Subtract : Sum  Inputs=+-
  Subtract1 : Sum
  Subtract2 : Sum  Inputs=-+
  Sum : Sum
  Sum1 : Sum
  φs_ref : Constant  Value=Motor_flux  SampleTime=Ts
  磁链PI : powerlib_extras/Discrete  Control Blocks/Discrete PI Controller  Kp=0.8  Ki=4  Par_Limits=[2 -2]  Init=0  Ts=Ts
  磁链PI1 : powerlib_extras/Discrete  Control Blocks/Discrete PI Controller  Commented=on  Kp=0.8  Ki=4  Par_Limits=[2 -2]  Init=0  Ts=Ts
  转矩pi : powerlib_extras/Discrete  Control Blocks/Discrete PI Controller  Kp=0.75  Ki=0.1  Par_Limits=[1000000 -1000000]  Init=0  Ts=Ts
  转矩pi1 : powerlib_extras/Discrete  Control Blocks/Discrete PI Controller  Commented=on  Kp=0.75  Ki=0.1  Par_Limits=[10000 -10000]  Init=0  Ts=Ts
  逆park变换 : ModelReference  ModelNameDialog=InvParkTran.slx  SimulationMode=Normal  ModelReferenceVersion=1.8
  速度pi1 : Subsystem  AncestorBlock=|  DialogController=POWERSYS.PowerSysDialog  mask(Discrete PI Controller){Kpw=0.0114, Kiw=0.019, Ba=0, Par_Limits=[34 -34], Init=0, Ts=Ts}
      | powerlib_extras/Discrete 
      | Control Blocks/Discrete
      | PI Controller
      mask prompts: Kpw "Proportional gain (Kp):"; Kiw "Integral gain (Ki):"; Ba "feedback gain (Ba)"; Par_Limits "Output limits: [ Upper   Lower ]"; Init "Output initial value:"; Ts "Sample time:"
      mask help: This block implements a discrete PI controller.
      mask init:
      | UpperLimit=Par_Limits(1);
      | LowerLimit=Par_Limits(2);
      | power_initmask();
      settings: LibrarySourceBlock=|
      | powerlib_extras/Discrete
      | Control Blocks/Discrete
      | PI Controller
      mask Help: This block is part of a subset of blocks in the Extras library that does not have documentation associated with it, other than the block mask description.
      mask Display: disp('PI');
  速度pi2 : Subsystem  Commented=on  AncestorBlock=|  DialogController=POWERSYS.PowerSysDialog  mask(Discrete PI Controller){Kpw=0.5, Kiw=120, Ba=0, Par_Limits=[1600 -1600], Init=0, Ts=Ts}
      | powerlib_extras/Discrete 
      | Control Blocks/Discrete
      | PI Controller
      mask prompts: Kpw "Proportional gain (Kp):"; Kiw "Integral gain (Ki):"; Ba "feedback gain (Ba)"; Par_Limits "Output limits: [ Upper   Lower ]"; Init "Output initial value:"; Ts "Sample time:"
      mask help: This block implements a discrete PI controller.
      mask init:
      | UpperLimit=Par_Limits(1);
      | LowerLimit=Par_Limits(2);
      | power_initmask();
      settings: LibrarySourceBlock=|
      | powerlib_extras/Discrete
      | Control Blocks/Discrete
      | PI Controller
      mask Help: This block is part of a subset of blocks in the Extras library that does not have documentation associated with it, other than the block mask description.
      mask Display: disp('PI');
  pulse : Outport
  wires:
  [Te] -> Subtract2/1
  Subtract/1 -> 速度pi1/1(Error)
  Sqrt/1 -> Subtract1/1
  speed/1 -> Subtract/1
  φs_ref/1 -> Subtract1/2
  [wm] -> Subtract/2
  Model1/1 -> pulse/1
  Subtract2/1 -> 转矩pi/1
  Subtract1/1 -> 磁链PI/1
  Sum/1 -> Square/1
  Constant/1 -> Sum/2
  [Motor_id] -> Gain/1
  [Motor_iq] -> Gain1/1
  Square1/1 -> Sum1/2
  Square/1 -> Sum1/1
  Sum1/1 -> Sqrt/1
  磁链PI/1 -> 逆park变换/1
  转矩pi/1 -> 逆park变换/2
  [theta] -> 逆park变换/3
  逆park变换/1 -> Model1/1
  逆park变换/2 -> Model1/2
  速度pi1/1(Out) -> Subtract2/2
  Gain/1 -> Sum/1
  Gain1/1 -> Square1/1

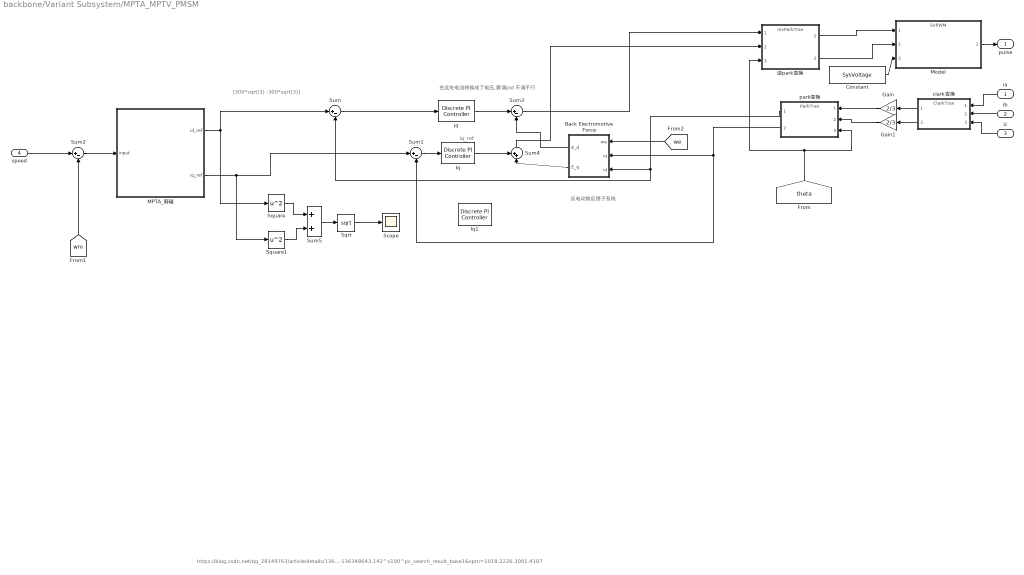
== system backbone/Variant Subsystem/MPTA_MPTV_PMSM ==
  note: [300*sqrt(3) -300*sqrt(3)]
  note: https://blog.csdn.net/qq_28149763/article/details/136348643?ops_request_misc=&request_id=&biz_id=102&utm_term=%E8%B6%85%E5%89%8D%E8%A7%92%E8%AE%A1%E7%AE%97MPTA&utm_medium=distribute.pc_search_result.none-task-blog-2~all~sobaiduweb~default-2-136348643.142^v100^pc_search_result_base1&spm=1018.2226.3001.4187
  note: iq_ref
  note: 反电动势反馈子系统
  note: 在此处电流转换成了电压,要调pid 不调不行
  ia : Inport
  ib : Inport  Port=2
  ic : Inport  Port=3
  speed : Inport  Port=4
  Back Electromotive Force : Subsystem
  Constant : Constant  Value=SysVoltage
  Gain : Gain  Gain=2/3
  Gain1 : Gain  Gain=2/3
  Id : powerlib_extras/Discrete  Control Blocks/Discrete PI Controller  Kp=50  Ki=0  Par_Limits=[300*sqrt(3) -300*sqrt(3)]  Init=0  Ts=Ts
  Iq : powerlib_extras/Discrete  Control Blocks/Discrete PI Controller  Kp=50  Ki=0  Par_Limits=[300*sqrt(3) -300*sqrt(3)]  Init=0  Ts=Ts
  Iq1 : powerlib_extras/Discrete  Control Blocks/Discrete PI Controller  Kp=0.1  Ki=0  Par_Limits=[SysVoltage*0.9*sqrt(3) -SysVoltage*0.9*sqrt(3)]  Init=0  Ts=Ts
  MPTA_弱磁 : Subsystem  Variant=on
  Model : ModelReference  ModelNameDialog=SVPWM.slx  SimulationMode=Normal  ModelReferenceVersion=1.9
  Scope : Scope
  Sqrt : Sqrt
  Square : Math  Operator=square
  Square1 : Math  Operator=square
  Sum{,1..3} (4 alike) : Sum  Inputs=|+-
  Sum4 : Sum  Inputs=++|
  Sum5 : Sum
  clark变换 : ModelReference  ModelNameDialog=ClarkTran.slx  SimulationMode=Normal  ModelReferenceVersion=1.13
  park变换 : ModelReference  ModelNameDialog=ParkTran.slx  SimulationMode=Normal  ModelReferenceVersion=1.9
  逆park变换 : ModelReference  ModelNameDialog=InvParkTran.slx  SimulationMode=Normal  ModelReferenceVersion=1.8
  pulse : Outport
  wires:
  Sum3/1 -> 逆park变换/1
  park变换/2 -> Back Electromotive Force/2(iq), Sum1/2
  Sum4/1 -> 逆park变换/2
  Back Electromotive Force/1(E_d) -> Sum3/2
  clark变换/2 -> Gain1/1
  ia/1 -> clark变换/1
  Square/1 -> Sum5/1
  Sqrt/1 -> Scope/1
  ic/1 -> clark变换/3
  ib/1 -> clark变换/2
  Sum1/1 -> Iq/1
  clark变换/1 -> Gain/1
  Iq/1 -> Sum4/1
  [theta] -> park变换/3, 逆park变换/3
  Back Electromotive Force/2(E_q) -> Sum4/2
  Id/1 -> Sum3/1
  Sum/1 -> Id/1
  park变换/1 -> Sum/2, Back Electromotive Force/3(id)
  [wm] -> Sum2/2
  逆park变换/2 -> Model/2
  speed/1 -> Sum2/1
  Square1/1 -> Sum5/2
  Model/1 -> pulse/1
  逆park变换/1 -> Model/1
  Gain/1 -> park变换/1
  Sum5/1 -> Sqrt/1
  [we] -> Back Electromotive Force/1(we)
  Gain1/1 -> park变换/2
  Sum2/1 -> MPTA_弱磁/1(input)
  MPTA_弱磁/2(iq_ref) -> Square1/1, Sum1/1
  MPTA_弱磁/1(id_ref) -> Sum/1, Square/1
  Constant/1 -> Model/3

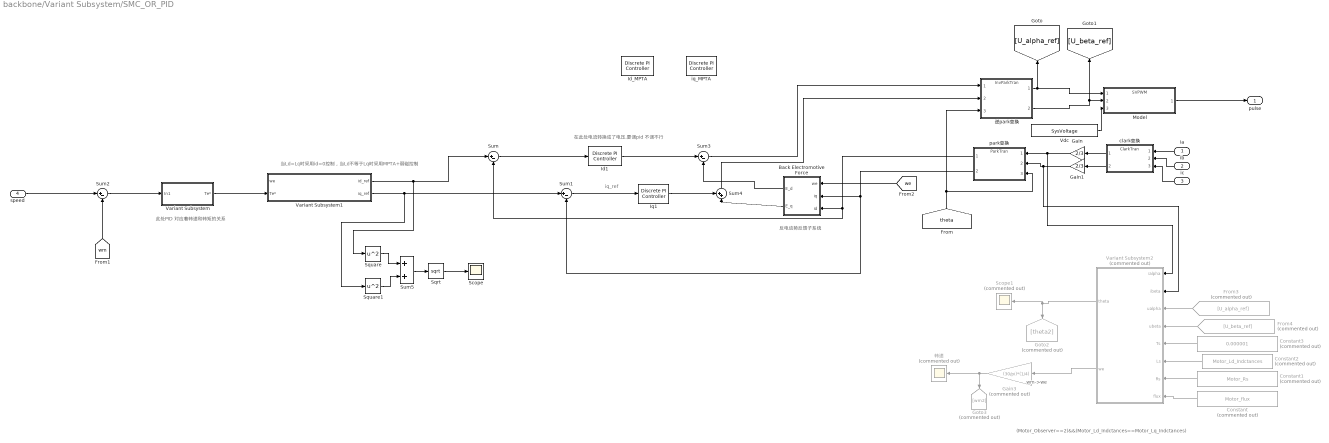
== system backbone/Variant Subsystem/SMC_OR_PID ==
  note: 当Ld=Lq时采用id=0控制，当Ld不等于Lq时采用MPTA+弱磁控制
  note: 此处PID 对应着转速和转矩的关系
  note: (Motor_Observer==2)&&(Motor_Ld_Indctances==Motor_Lq_Indctances)
  note: 在此处电流转换成了电压,要调pid 不调不行
  note: wm->we
  note: iq_ref
  note: 反电动势反馈子系统
  ia : Inport
  ib : Inport  Port=2
  ic : Inport  Port=3
  speed : Inport  Port=4
  Back Electromotive Force : Subsystem
  Constant : Constant  Commented=on  Value=Motor_flux
  Constant1 : Constant  Commented=on  Value=Motor_Rs
  Constant2 : Constant  Commented=on  Value=Motor_Ld_Indctances
  Constant3 : Constant  Commented=on  Value=0.000001
  From3 : From  Commented=on  GotoTag=U_alpha_ref
  From4 : From  Commented=on  GotoTag=U_beta_ref
  Gain : Gain  Gain=2/3
  Gain1 : Gain  Gain=2/3
  Gain3 : Gain  Commented=on  Gain=(30/pi)*(1/4)
  Goto2 : Goto  Commented=on  GotoTag=theta2
  Goto3 : Goto  Commented=on  GotoTag=wm2
  Id1 : powerlib_extras/Discrete  Control Blocks/Discrete PI Controller  Kp=133  Ki=0  Par_Limits=[SysVoltage*sqrt(3) -SysVoltage*sqrt(3)]  Init=0  Ts=1e-5
  Id_MPTA : powerlib_extras/Discrete  Control Blocks/Discrete PI Controller  Kp=50  Ki=250  Par_Limits=[4000 -4000]  Init=0  Ts=Ts
  Iq1 : powerlib_extras/Discrete  Control Blocks/Discrete PI Controller  Kp=133  Ki=0  Par_Limits=[SysVoltage*sqrt(3) -SysVoltage*sqrt(3)]  Init=0  Ts=1e-5
  Model : ModelReference  ModelNameDialog=SVPWM.slx  SimulationMode=Normal  ModelReferenceVersion=1.9
  Scope : Scope
  Scope1 : Scope  Commented=on
  Sqrt : Sqrt
  Square : Math  Operator=square
  Square1 : Math  Operator=square
  Sum{,1..3} (4 alike) : Sum  Inputs=|+-
  Sum4 : Sum  Inputs=++|
  Sum5 : Sum
  Variant Subsystem : Subsystem  Variant=on
  Variant Subsystem1 : Subsystem  Variant=on
  Variant Subsystem2 : Subsystem  Commented=on  Variant=on
  Vdc : Constant  Value=SysVoltage
  clark变换 : ModelReference  ModelNameDialog=ClarkTran.slx  SimulationMode=Normal  ModelReferenceVersion=1.13
  iq_MPTA : powerlib_extras/Discrete  Control Blocks/Discrete PI Controller  Kp=50  Ki=250  Par_Limits=[4000 -4000]  Init=0  Ts=Ts
  park变换 : ModelReference  ModelNameDialog=ParkTran.slx  SimulationMode=Normal  ModelReferenceVersion=1.9
  转速 : Scope  Commented=on
  逆park变换 : ModelReference  ModelNameDialog=InvParkTran.slx  SimulationMode=Normal  ModelReferenceVersion=1.8
  pulse : Outport
  wires:
  Sum1/1 -> Iq1/1
  speed/1 -> Sum2/1
  Sum/1 -> Id1/1
  [theta] -> park变换/3, 逆park变换/3
  Sum4/1 -> 逆park变换/2
  Sum3/1 -> 逆park变换/1
  clark变换/2 -> Gain1/1
  park变换/1 -> Back Electromotive Force/3(id), Sum/2
  clark变换/1 -> Gain/1
  park变换/2 -> Sum1/2, Back Electromotive Force/2(iq)
  Model/1 -> pulse/1
  ia/1 -> clark变换/1
  ib/1 -> clark变换/2
  ic/1 -> clark变换/3
  Iq1/1 -> Sum4/1
  Id1/1 -> Sum3/1
  Sum2/1 -> Variant Subsystem/1(In1)
  Variant Subsystem/1(Te*) -> Variant Subsystem1/2(Te*)
  Back Electromotive Force/2(E_q) -> Sum4/2
  Back Electromotive Force/1(E_d) -> Sum3/2
  [we] -> Back Electromotive Force/1(we)
  Variant Subsystem1/2(iq_ref) -> Square1/1, Sum1/1
  Variant Subsystem1/1(id_ref) -> Square/1, Sum/1
  Constant3/1 -> Variant Subsystem2/5(Ts)
  Constant2/1 -> Variant Subsystem2/6(Ls)
  Constant1/1 -> Variant Subsystem2/7(Rs)
  Constant/1 -> Variant Subsystem2/8(flux)
  Variant Subsystem2/2(we) -> Gain3/1
  From4/1 -> Variant Subsystem2/4(ubeta)
  From3/1 -> Variant Subsystem2/3(ualpha)
  Variant Subsystem2/1(theta) -> Scope1/1, Goto2/1
  Gain3/1 -> Goto3/1, 转速/1
  逆park变换/1 -> Model/1, [U_alpha_ref]
  逆park变换/2 -> Model/2, [U_beta_ref]
  Gain/1 -> Variant Subsystem2/1(ialpha), park变换/1
  Gain1/1 -> Variant Subsystem2/2(ibeta), park变换/2
  Square/1 -> Sum5/1
  Square1/1 -> Sum5/2
  Sum5/1 -> Sqrt/1
  Sqrt/1 -> Scope/1
  Vdc/1 -> Model/3
  [wm] -> Sum2/2

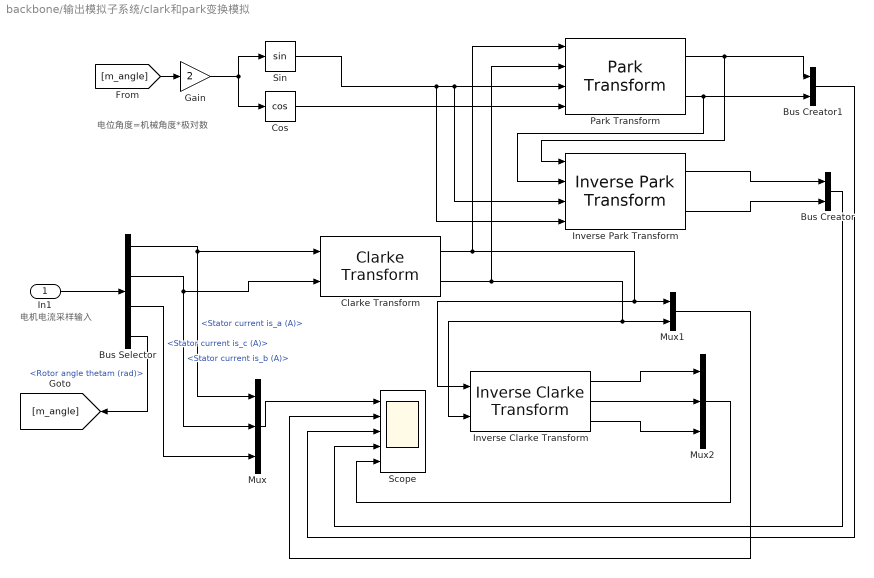
== system backbone/输出模拟子系统/clark和park变换模拟 ==
  note: 电位角度=机械角度*极对数
  note: 电机电流采样输入
  In1 : Inport
  Bus Creator : BusCreator  Inputs=2
  Bus Creator1 : BusCreator  Inputs=2
  Bus Selector : BusSelector  OutputSignals=Stator current is_a (A),Stator current is_b (A),Stator current is_c (A),Rotor angle thetam (rad)
  Clarke Transform : mcbcontrolslib/Clarke Transform  VariantControl=Variant2
      settings: LibrarySourceBlock=mcblib/Controls/Math Transforms/Clarke Transform
  Cos : Trigonometry  Operator=cos
  Gain : Gain  Gain=2
  Inverse Clarke Transform : mcbcontrolslib/Inverse Clarke Transform
      settings: LibrarySourceBlock=mcblib/Controls/Math Transforms/Inverse Clarke Transform
  Inverse Park Transform : mcbcontrolslib/Inverse Park Transform  AxisAlignment=D-axis
      settings: LibrarySourceBlock=mcbhdllib/Controls/Math Transforms/Inverse Park Transform
  Mux : Mux  Inputs=3
  Mux1 : Mux  Inputs=2
  Mux2 : Mux  Inputs=3
  Park Transform : mcbcontrolslib/Park Transform  AxisAlignment=D-axis
      settings: LibrarySourceBlock=mcbhdllib/Controls/Math Transforms/Park Transform
  Scope : Scope  NumInputPorts=5
  Sin : Trigonometry
  wires:
  In1/1 -> Bus Selector/1
  Clarke Transform/1 -> Park Transform/1, Inverse Clarke Transform/1, Mux1/1
  Clarke Transform/2 -> Park Transform/2, Inverse Clarke Transform/2, Mux1/2
  Mux1/1 -> Scope/2
  Bus Selector/1 -> Mux/1, Clarke Transform/1  "<Stator current is_a (A)>"
  Bus Selector/2 -> Mux/2, Clarke Transform/2  "<Stator current is_b (A)>"
  Mux/1 -> Scope/1
  Bus Selector/3 -> Mux/3  "<Stator current is_c (A)>"
  Mux2/1 -> Scope/5
  Inverse Clarke Transform/1 -> Mux2/1
  Inverse Clarke Transform/2 -> Mux2/2
  Inverse Clarke Transform/3 -> Mux2/3
  Bus Selector/4 -> [m_angle]  "<Rotor angle thetam (rad)>"
  [m_angle] -> Gain/1
  Gain/1 -> Sin/1, Cos/1
  Cos/1 -> Park Transform/4
  Sin/1 -> Inverse Park Transform/4, Inverse Park Transform/3, Park Transform/3
  Park Transform/1 -> Inverse Park Transform/1, Bus Creator1/1
  Park Transform/2 -> Inverse Park Transform/2, Bus Creator1/2
  Inverse Park Transform/1 -> Bus Creator/1
  Inverse Park Transform/2 -> Bus Creator/2
  Bus Creator1/1 -> Scope/3
  Bus Creator/1 -> Scope/4

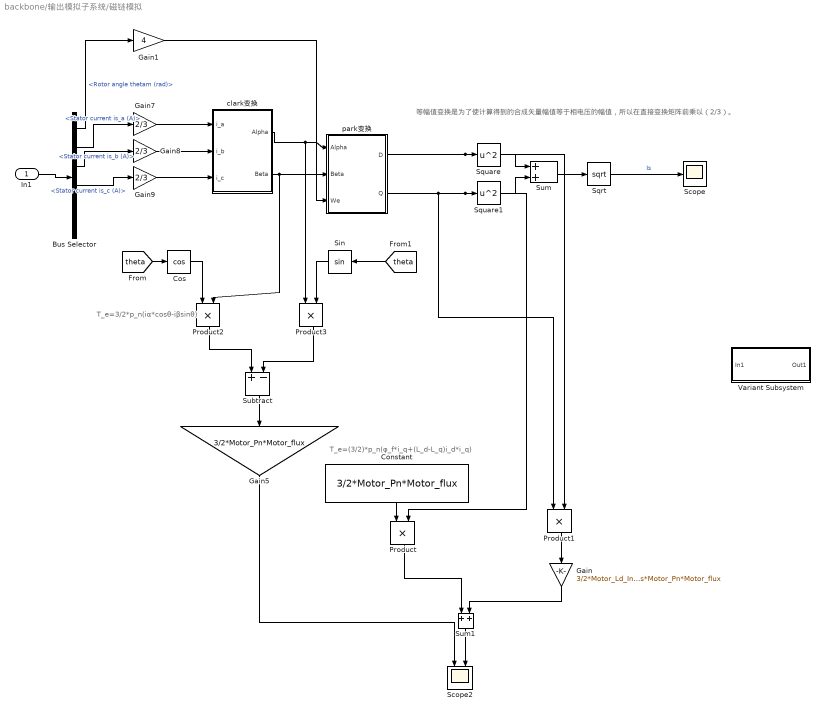
== system backbone/输出模拟子系统/磁链模拟 ==
  note: T_e=3/2*p_n(iα*cosθ-iβsinθ)
  note: 等幅值变换是为了使计算得到的合成矢量幅值等于相电压的幅值，所以在直接变换矩阵前乘以（2/3）。
  note: T_e=(3/2)*p_n(φ_f*i_q+(L_d-L_q)i_d*i_q)
  In1 : Inport
  Bus Selector : BusSelector  OutputSignals=Rotor angle thetam (rad),Stator current is_a (A),Stator current is_b (A),Stator current is_c (A),Electromagnetic torque Te (N*m),Rotor speed wm (rad/s)
  Constant : Constant  Value=3/2*Motor_Pn*Motor_flux
  Cos : Trigonometry  Operator=cos
  Gain : Gain  Gain=3/2*Motor_Ld_Indctances*Motor_Lq_Indctances*Motor_Pn*Motor_flux
  Gain1 : Gain  Gain=4
  Gain5 : Gain  Gain=3/2*Motor_Pn*Motor_flux
  Gain7 : Gain  Gain=2/3
  Gain8 : Gain  Gain=2/3
  Gain9 : Gain  Gain=2/3
  Product{,1..3} (4 alike) : Product
  Scope : Scope
  Scope2 : Scope  NumInputPorts=2
  Sin : Trigonometry
  Sqrt : Sqrt
  Square : Math  Operator=square
  Square1 : Math  Operator=square
  Subtract : Sum  Inputs=+-
  Sum : Sum
  Sum1 : Sum
  Variant Subsystem : Subsystem  Variant=on
  clark变换 : Subsystem
  park变换 : Subsystem
  wires:
  In1/1 -> Bus Selector/1
  Bus Selector/2 -> Gain7/1  "<Stator current is_a (A)>"
  Bus Selector/3 -> Gain8/1  "<Stator current is_b (A)>"
  Bus Selector/4 -> Gain9/1  "<Stator current is_c (A)>"
  Constant/1 -> Product/1
  clark变换/1(Alpha) -> park变换/1(Alpha), Product3/1
  clark变换/2(Beta) -> Product2/2, park变换/2(Beta)
  Bus Selector/1 -> Gain1/1  "<Rotor angle thetam (rad)>"
  Gain1/1 -> park变换/3(We)
  Square/1 -> Sum/1
  Square1/1 -> Sum/2
  Sum/1 -> Sqrt/1
  Sqrt/1 -> Scope/1  "Is"
  Product1/1 -> Gain/1
  Product/1 -> Sum1/1
  Gain/1 -> Sum1/2
  Sum1/1 -> Scope2/2
  park变换/1(D) -> Product1/2, Square/1
  park变换/2(Q) -> Product/2, Square1/1, Product1/1
  [theta] -> Cos/1
  Cos/1 -> Product2/1
  [theta] -> Sin/1
  Sin/1 -> Product3/2
  Product2/1 -> Subtract/1
  Product3/1 -> Subtract/2
  Subtract/1 -> Gain5/1
  Gain7/1 -> clark变换/1(i_a)
  Gain8/1 -> clark变换/2(i_b)
  Gain9/1 -> clark变换/3(i_c)
  Gain5/1 -> Scope2/1

== system backbone/Variant Subsystem/BangBang_PMSM/Speed ==
  note: Pierre Giroux, Gilbert Sybille
      | Power System Simulation Laboratory
      | IREQ, Hydro-Quebc
  note: Discrete PID Controller
  Error : Inport  SampleTime=Ts
  Discrete-Time Integrator : DiscreteIntegrator  InitialCondition=Init  SampleTime=Ts  LimitOutput=on  UpperSaturationLimit=UpperLimit  LowerSaturationLimit=LowerLimit  ICPrevOutput=DiscIntNeverNeededParam  ICPrevScaledInput=DiscIntNeverNeededParam
  Kp1 : Gain  Gain=Ba  SaturateOnIntegerOverflow=on  SampleTime=Ts  OutDataTypeStr=Inherit: Same as input  ParamDataTypeStr=Inherit: Same as input
  Kp4 : Gain  Gain=Kpw  SaturateOnIntegerOverflow=on  SampleTime=Ts  OutDataTypeStr=Inherit: Same as input  ParamDataTypeStr=Inherit: Same as input
  Kp5 : Gain  Gain=Kiw  SaturateOnIntegerOverflow=on  SampleTime=Ts  OutDataTypeStr=Inherit: Same as input  ParamDataTypeStr=Inherit: Same as input
  Saturation2 : Saturate  UpperLimit=UpperLimit  LowerLimit=LowerLimit  SampleTime=Ts
  Sum6 : Sum  Inputs=++-  InputSameDT=on  SaturateOnIntegerOverflow=on  SampleTime=Ts  OutDataTypeStr=Inherit: Same as first input
  Zero-Order Hold : ZeroOrderHold  SampleTime=Ts
  Out : Outport  SampleTime=Ts  InitialOutput=0
  wires:
  Kp1/1 -> Sum6/3
  Sum6/1 -> Saturation2/1
  Kp5/1 -> Discrete-Time Integrator/1
  Kp4/1 -> Zero-Order Hold/1
  Discrete-Time Integrator/1 -> Sum6/2
  Saturation2/1 -> Out/1
  Zero-Order Hold/1 -> Sum6/1
  Error/1 -> Kp4/1, Kp5/1, Kp1/1
